simulink model "Zarud_ZPT"  (R2018b)
settings: Solver=ode8  StartTime=0.0  StopTime=5  RelTol=1e-3
undefined symbols (not defined in the file): C, C_zpt_c, C_zpt_r, R_zarud
libraries: powerlib x7
settings Model: Creator=Anton  LastModifiedBy=VID Company
settings SFSimCC: SimUseLocalCustomCode=off
settings RTWCC: RTWUseLocalCustomCode=off
settings CodeAppCC: StateflowObjectComments=on
settings SimscapeCC: SimscapeNormalizeSystem=off

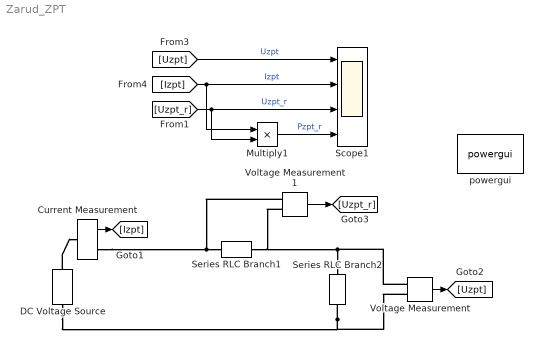
== system Zarud_ZPT ==
  Current Measurement : powerlib/Measurements/Current Measurement  PhasorSimulation=off  OutputType=Complex  PSBequivalent=0
  DC Voltage Source : powerlib/Electrical Sources/DC Voltage Source  Amplitude=690  Measurements=None
  Multiply1 : Product
  Scope1 : Scope  NumInputPorts=4
  Series RLC Branch1 : powerlib/Elements/Series RLC Branch  LConnTagsString=__new0  RConnTagsString=__new0  BranchType=R  Resistance=R_zarud  Inductance=250e-6  SetiL0=off  InitialCurrent=0  Capacitance=C  Setx0=on  InitialVoltage=U  Measurements=None
  Series RLC Branch2 : powerlib/Elements/Series RLC Branch  LConnTagsString=__new0  RConnTagsString=__new0  BranchType=RC  Resistance=C_zpt_r  Inductance=250e-6  SetiL0=off  InitialCurrent=0  Capacitance=C_zpt_c  Setx0=on  InitialVoltage=0  Measurements=None
  Voltage Measurement : powerlib/Measurements/Voltage Measurement  PhasorSimulation=off  OutputType=Complex  PSBequivalent=0
  Voltage Measurement1 : powerlib/Measurements/Voltage Measurement  PhasorSimulation=off  OutputType=Complex  PSBequivalent=0
  powergui : powerlib/powergui  Priority=1  SimulationMode=Discrete  SampleTime=1e-6  frequency=60  Iterations=50  frequencyindice=0  Pbase=100e6  ErrMax=1e-4  UnitsV=kV  UnitsW=MW  buscounter=0  FunctionMessages=off  echomessages=off  EnableUseOfTLC=off  CurrentSourceSwitches=off  DisableSnubberDevices=off  DisableRonSwitches=off  DisableVfSwitches=off  DisplayEquations=off  SolverType=Tustin/Backward Euler (TBE)  Interpol=off  ExternalGateDelay=off  methode=off  Ts=100  x0status=blocks  SPID=off  SwTol=0  HookPort=off  RestoreLinks=warning  ResistiveCurrentMeasurement=off  Frange=[0:2:500]  Ylog=off  Xlog=on  ShowGrid=off  save=off  variable=ZData  structure=0  ZoomFFT=off  StartTime=0.0  cycles=1  DisplayStyle=1  fundamental=60  FreqAxis=off  MaxFrequency=1000  frequencyindicesteady=1  RmsSteady=1  display=off
  wires:
  Voltage Measurement/1 -> [Uzpt]
  [Izpt] -> Scope1/2, Multiply1/1  "Izpt"
  [Uzpt] -> Scope1/1  "Uzpt"
  Current Measurement/1 -> [Izpt]
  Voltage Measurement1/1 -> [Uzpt_r]
  [Uzpt_r] -> Scope1/3, Multiply1/2  "Uzpt_r"
  Multiply1/1 -> Scope1/4  "Pzpt_r"
  connections:
  Series RLC Branch2/RConn1 -- DC Voltage Source/LConn1 -- Voltage Measurement/LConn2
  Current Measurement/RConn1 -- Voltage Measurement1/LConn1 -- Series RLC Branch1/LConn1
  DC Voltage Source/RConn1 -- Current Measurement/LConn1
  Voltage Measurement/LConn1 -- Voltage Measurement1/LConn2 -- Series RLC Branch1/RConn1 -- Series RLC Branch2/LConn1
